simulink model "Prob8"  (R2020b)
settings: Solver=VariableStepAuto  StartTime=0.0  StopTime=10.0  RelTol=1e-3
settings Model: Creator=shoun  LastModifiedBy=shoun

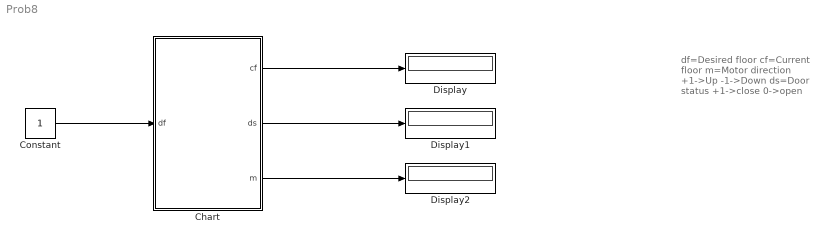
== system Prob8 ==
  note: df=Desired floor
      | cf=Current floor
      | m=Motor direction
      | +1->Up
      | -1->Down
      | ds=Door status
      | +1->close
      | 0->open
  Chart : Stateflow chart  TreatAsAtomicUnit=on
  Constant : Constant
  Display : Display
  Display1 : Display
  Display2 : Display
  wires:
  Chart/1(cf) -> Display/1
  Chart/2(ds) -> Display1/1
  Chart/3(m) -> Display2/1
  Constant/1 -> Chart/1(df)

== stateflow chart Prob8/Chart ==
  state Lift
    state Idle
      entry:m=0;
    state Door_closed
      entry:ds=1;
    state Down
      entry:m=-1;
      during:cf=cf-1;
    state Up
      entry:m=1;
      during:cf=cf+1;
    state Stop
      entry:m=0;ds=1;
      during:m=0;
    state Door_open
      entry:ds=0;
      during:ds=0;m=0;
    (default) -> Idle
    Idle -> Idle [order 2] : [df==cf]
    Door_open -> Idle : after(2,sec)
    Idle -> Door_closed [order 1] : [df~=cf]
    Door_closed -> Up [order 1] : [df>cf]
    Door_closed -> Down [order 2] : [df<cf]
    Down -> Stop : [df==cf]
    Up -> Stop : [df==cf]
    Stop -> Door_open : [df==cf]
  (default) -> Lift
  data: cf output =0; df input; ds output; m output
